simulink model "sampleModel2071"  (R2023a)
settings: Solver=VariableStepAuto  StartTime=0.0  StopTime=10.0  RelTol=1e-3
libraries: hdlsllib x7, simulink x1
settings Model: Creator=user1  LastModifiedBy=user1

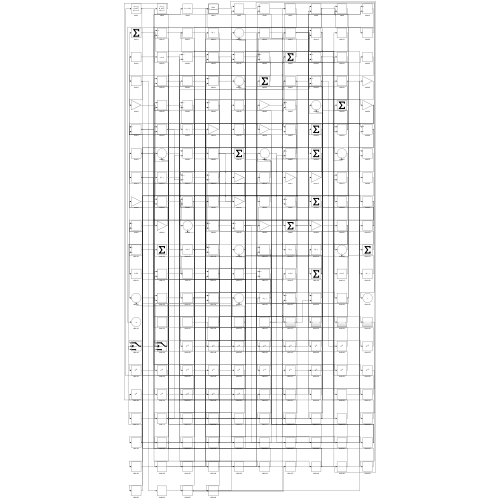
[thumbnail: Simulink's stored preview of the top-level diagram]
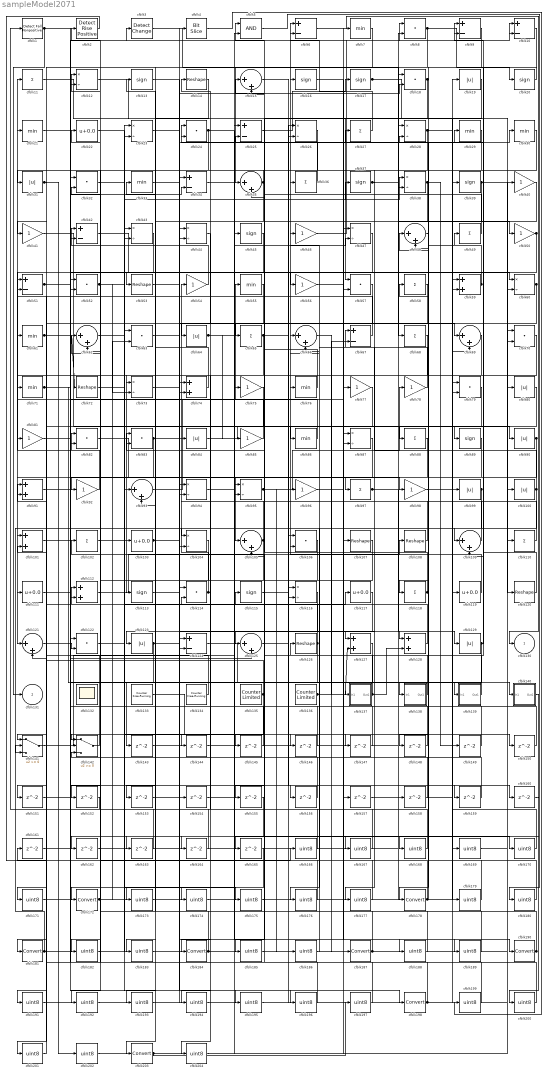
== system sampleModel2071 ==
  cfblk1 : hdlsllib/Logic and Bit Operations/Detect Fall Nonpositive  vinit=0  OutDataTypeStr=boolean
  cfblk{6,9..10,25,34,42,51,67,124} (9 alike) : Sum  Inputs=+-
  cfblk{19,31,64,80,84,90,99..100,123,129} (10 alike) : Abs  SaturateOnIntegerOverflow=off
  cfblk{59,74,91,101,112,127..128} (7 alike) : Sum
  cfblk{11,27,36,49,58,65,68,88,97,102,110,118} (12 alike) : Sum  Inputs=+
  cfblk{22,103,111,117,119} (5 alike) : Bias  Bias=0.0  SaturateOnIntegerOverflow=off
  cfblk{12,23,26,28,38,43..44,47,60,73,87,94..95,104,116} (15 alike) : Product  Inputs=*/  RndMeth=Zero  SaturateOnIntegerOverflow=on
  cfblk{15,35,48,62,66,69,93,105,109,121,125} (11 alike) : Sum  Inputs=|++
  cfblk{8,18,24,32,52,57,63,70,79,82..83,106,114,122} (14 alike) : DotProduct  OutDataTypeStr=Inherit: Inherit via internal rule
  cfblk{14,53,72,107..108,120,126} (7 alike) : Reshape
  cfblk{13,16..17,20,37,39,45,89,113,115} (10 alike) : Signum
  cfblk132 : Scope
      settings: Floating=on
  cfblk133 : hdlsllib/Sources/Counter Free-Running  NumBits=16  tsamp=-1
  cfblk134 : hdlsllib/Sources/Counter Free-Running  NumBits=16  tsamp=-1
  cfblk135 : hdlsllib/Sources/Counter Limited  uplimit=7  tsamp=-1
  cfblk136 : hdlsllib/Sources/Counter Limited  uplimit=7  tsamp=-1
  cfblk137 : Subsystem
      settings: LibrarySourceBlock=|
      | hdlsllib/Ports &
      | Subsystems/Subsystem
  cfblk138 : Subsystem
      settings: LibrarySourceBlock=|
      | hdlsllib/Ports &
      | Subsystems/Subsystem
  cfblk139 : Subsystem
      settings: LibrarySourceBlock=|
      | hdlsllib/Ports &
      | Subsystems/Subsystem
  cfblk140 : Subsystem
      settings: LibrarySourceBlock=|
      | hdlsllib/Ports &
      | Subsystems/Subsystem
  cfblk141 : Switch  SaturateOnIntegerOverflow=off  InputSameDT=off
  cfblk142 : Switch  SaturateOnIntegerOverflow=off  InputSameDT=off
  cfblk{143..165} (23 alike) : Delay  SampleTime=1
  cfblk{166..171,173..177,179..180,182..183,185..186,188..189,191..197,199..202,204} (31 alike) : DataTypeConversion  OutDataTypeStr=uint8  SaturateOnIntegerOverflow=off  RndMeth=Floor
  cfblk{172,178,181,184,187,190,198,203} (8 alike) : DataTypeConversion  SaturateOnIntegerOverflow=off  RndMeth=Floor
  cfblk2 : hdlsllib/Logic and Bit Operations/Detect Rise Positive  vinit=0  OutDataTypeStr=boolean
  cfblk{7,21,29..30,33,55,61,71,76,86} (10 alike) : MinMax
  cfblk3 : simulink/Logic and Bit Operations/Detect Change  vinit=0  OutDataTypeStr=boolean
      settings: LibrarySourceBlock=|
      | hdlsllib/Logic and Bit
      | Operations/Detect
      | Change
  cfblk4 : hdlsllib/Logic and Bit Operations/Bit Slice  lidx=7  ridx=0
  cfblk{40..41,46,50,54,56,75,77..78,81,85,92,96,98} (14 alike) : Gain
  cfblk5 : Logic  AllPortsSameDT=off  OutDataTypeStr=boolean
  cfblk130 : Outport  VectorParamsAs1DForOutWhenUnconnected=off
  cfblk131 : Outport  Port=2  VectorParamsAs1DForOutWhenUnconnected=off
  wires:
  cfblk112/1 -> cfblk108/1
  cfblk19/1 -> cfblk57/1
  cfblk129/1 -> cfblk9/2, cfblk164/1
  cfblk20/1 -> cfblk35/1
  cfblk18/1 -> cfblk118/1, cfblk65/1
  cfblk86/1 -> cfblk55/1
  cfblk90/1 -> cfblk112/1, cfblk104/2
  cfblk67/1 -> cfblk11/1
  cfblk46/1 -> cfblk8/1
  cfblk71/1 -> cfblk140/1(In1), cfblk125/2
  cfblk114/1 -> cfblk54/1, cfblk174/1
  cfblk69/1 -> cfblk113/1
  cfblk36/1 -> cfblk6/1
  cfblk95/1 -> cfblk78/1, cfblk27/1, cfblk165/1, cfblk186/1
  cfblk43/1 -> cfblk121/1
  cfblk100/1 -> cfblk38/1, cfblk109/2, cfblk67/1
  cfblk119/1 -> cfblk16/1
  cfblk45/1 -> cfblk53/1
  cfblk76/1 -> cfblk35/2
  cfblk103/1 -> cfblk34/1, cfblk18/2
  cfblk53/1 -> cfblk114/1
  cfblk123/1 -> cfblk74/1, cfblk128/1, cfblk142/2
  cfblk121/1 -> cfblk122/2
  cfblk56/1 -> cfblk30/1
  cfblk87/1 -> cfblk111/1
  cfblk28/1 -> cfblk127/1, cfblk60/1
  cfblk15/1 -> cfblk88/1
  cfblk70/1 -> cfblk181/1
  cfblk44/1 -> cfblk64/1
  cfblk66/1 -> cfblk187/1
  cfblk82/1 -> cfblk98/1
  cfblk109/1 -> cfblk58/1
  cfblk59/1 -> cfblk49/1, cfblk36/1
  cfblk8/1 -> cfblk123/1, cfblk82/2, cfblk20/1
  cfblk26/1 -> cfblk172/1
  cfblk92/1 -> cfblk21/1
  cfblk89/1 -> cfblk105/1
  cfblk27/1 -> cfblk6/2
  cfblk10/1 -> cfblk89/1
  cfblk75/1 -> cfblk203/1
  cfblk142/1 -> cfblk51/1
  cfblk42/1 -> cfblk107/1
  cfblk1/1 -> cfblk131/1, cfblk59/2
  cfblk6/1 -> cfblk130/1
  cfblk134/1 -> cfblk82/1
  cfblk35/1 -> cfblk31/1, cfblk163/1
  cfblk126/1 -> cfblk91/1, cfblk33/1, cfblk194/1
  cfblk52/1 -> cfblk93/1, cfblk73/2
  cfblk72/1 -> cfblk103/1
  cfblk64/1 -> cfblk85/1, cfblk47/2, cfblk167/1
  cfblk94/1 -> cfblk190/1
  cfblk141/1 -> cfblk45/1
  cfblk11/1 -> cfblk119/1
  cfblk47/1 -> cfblk74/2
  cfblk139/1(Out1) -> cfblk102/1
  cfblk7/1 -> cfblk41/1
  cfblk54/1 -> cfblk42/1
  cfblk41/1 -> cfblk110/1
  cfblk110/1 -> cfblk5/1
  cfblk97/1 -> cfblk10/1, cfblk129/1
  cfblk73/1 -> cfblk29/1
  cfblk60/1 -> cfblk92/1, cfblk109/1
  cfblk93/1 -> cfblk7/1
  cfblk12/1 -> cfblk80/1
  cfblk78/1 -> cfblk51/2
  cfblk39/1 -> cfblk120/1, cfblk73/1
  cfblk24/1 -> cfblk43/2, cfblk87/2
  cfblk9/1 -> cfblk138/1(In1)
  cfblk128/1 -> cfblk12/1
  cfblk83/1 -> cfblk90/1, cfblk171/1
  cfblk105/1 -> cfblk84/1, cfblk204/1
  cfblk137/1(Out1) -> cfblk96/1, cfblk128/2
  cfblk65/1 -> cfblk104/1, cfblk15/2, cfblk139/1(In1), cfblk155/1
  cfblk74/1 -> cfblk13/1
  cfblk85/1 -> cfblk61/1
  cfblk37/1 -> cfblk9/1, cfblk97/1
  cfblk106/1 -> cfblk184/1
  cfblk113/1 -> cfblk38/2
  cfblk118/1 -> cfblk15/1, cfblk83/1
  cfblk108/1 -> cfblk14/1
  cfblk17/1 -> cfblk99/1, cfblk69/2, cfblk50/1
  cfblk25/1 -> cfblk17/1
  cfblk84/1 -> cfblk86/1
  cfblk49/1 -> cfblk25/2
  cfblk136/1 -> cfblk127/2, cfblk67/2
  cfblk48/1 -> cfblk178/1
  cfblk61/1 -> cfblk72/1, cfblk95/2
  cfblk29/1 -> cfblk44/2
  cfblk32/1 -> cfblk198/1
  cfblk3/1 -> cfblk68/1
  cfblk96/1 -> cfblk47/1
  cfblk50/1 -> cfblk57/2, cfblk173/1, cfblk177/1
  cfblk124/1 -> cfblk137/1(In1)
  cfblk55/1 -> cfblk101/1
  cfblk102/1 -> cfblk37/1
  cfblk138/1(Out1) -> cfblk46/1
  cfblk104/1 -> cfblk124/2
  cfblk122/1 -> cfblk117/1
  cfblk135/1 -> cfblk142/1, cfblk91/2
  cfblk120/1 -> cfblk24/1
  cfblk21/1 -> cfblk3/1
  cfblk99/1 -> cfblk141/3, cfblk176/1
  cfblk23/1 -> cfblk4/1
  cfblk91/1 -> cfblk34/2
  cfblk51/1 -> cfblk10/2, cfblk160/1
  cfblk38/1 -> cfblk125/1, cfblk149/1
  cfblk57/1 -> cfblk141/1
  cfblk31/1 -> cfblk71/1, cfblk202/1
  cfblk13/1 -> cfblk69/1
  cfblk111/1 -> cfblk76/1
  cfblk34/1 -> cfblk56/1
  cfblk127/1 -> cfblk143/1
  cfblk143/1 -> cfblk28/1
  cfblk68/1 -> cfblk144/1
  cfblk144/1 -> cfblk5/2
  cfblk58/1 -> cfblk145/1
  cfblk145/1 -> cfblk93/2
  cfblk63/1 -> cfblk146/1
  cfblk146/1 -> cfblk25/1
  cfblk22/1 -> cfblk147/1
  cfblk147/1 -> cfblk43/1
  cfblk30/1 -> cfblk148/1
  cfblk148/1 -> cfblk44/1
  cfblk149/1 -> cfblk18/1
  cfblk125/1 -> cfblk150/1
  cfblk150/1 -> cfblk122/1
  cfblk80/1 -> cfblk151/1
  cfblk151/1 -> cfblk12/2
  cfblk107/1 -> cfblk152/1
  cfblk152/1 -> cfblk1/1
  cfblk14/1 -> cfblk153/1
  cfblk101/1 -> cfblk156/1
  cfblk156/1 -> cfblk105/2
  cfblk157/1 -> cfblk79/1
  cfblk158/1 -> cfblk142/3
  cfblk115/1 -> cfblk159/1
  cfblk159/1 -> cfblk24/2
  cfblk161/1 -> cfblk52/2
  cfblk140/1(Out1) -> cfblk162/1
  cfblk162/1 -> cfblk8/2
  cfblk163/1 -> cfblk121/2
  cfblk164/1 -> cfblk23/1
  cfblk2/1 -> cfblk166/1
  cfblk166/1 -> cfblk22/1
  cfblk167/1 -> cfblk2/1
  cfblk40/1 -> cfblk168/1
  cfblk168/1 -> cfblk114/2
  cfblk98/1 -> cfblk169/1
  cfblk169/1 -> cfblk40/1
  cfblk154/1 -> cfblk170/1
  cfblk170/1 -> cfblk59/1
  cfblk171/1 -> cfblk154/1
  cfblk172/1 -> cfblk158/1, cfblk157/1, cfblk63/2
  cfblk173/1 -> cfblk26/1
  cfblk174/1 -> cfblk26/2
  cfblk62/1 -> cfblk175/1
  cfblk175/1 -> cfblk79/2
  cfblk176/1 -> cfblk62/1
  cfblk177/1 -> cfblk62/2
  cfblk178/1 -> cfblk63/1, cfblk28/2
  cfblk133/1 -> cfblk179/1
  cfblk179/1 -> cfblk48/1
  cfblk5/1 -> cfblk180/1
  cfblk180/1 -> cfblk48/2
  cfblk181/1 -> cfblk95/1, cfblk141/2, cfblk23/2
  cfblk155/1 -> cfblk182/1
  cfblk182/1 -> cfblk70/1
  cfblk117/1 -> cfblk183/1
  cfblk183/1 -> cfblk70/2
  cfblk184/1 -> cfblk42/2, cfblk124/1
  cfblk88/1 -> cfblk185/1
  cfblk185/1 -> cfblk106/1
  cfblk186/1 -> cfblk106/2
  cfblk187/1 -> cfblk112/2, cfblk19/1
  cfblk33/1 -> cfblk188/1
  cfblk188/1 -> cfblk66/1
  cfblk16/1 -> cfblk189/1
  cfblk189/1 -> cfblk66/2
  cfblk190/1 -> cfblk83/2, cfblk87/1, cfblk126/1
  cfblk79/1 -> cfblk191/1
  cfblk191/1 -> cfblk94/1
  cfblk165/1 -> cfblk192/1
  cfblk192/1 -> cfblk94/2
  cfblk116/1 -> cfblk193/1
  cfblk193/1 -> cfblk39/1
  cfblk194/1 -> cfblk116/1
  cfblk153/1 -> cfblk195/1
  cfblk195/1 -> cfblk116/2
  cfblk81/1 -> cfblk196/1
  cfblk196/1 -> cfblk115/1
  cfblk197/1 -> cfblk81/1
  cfblk198/1 -> cfblk60/2, cfblk101/2, cfblk52/1
  cfblk4/1 -> cfblk199/1
  cfblk199/1 -> cfblk32/1
  cfblk160/1 -> cfblk200/1
  cfblk200/1 -> cfblk32/2
  cfblk77/1 -> cfblk201/1
  cfblk201/1 -> cfblk161/1
  cfblk202/1 -> cfblk77/1
  cfblk203/1 -> cfblk197/1, cfblk100/1
  cfblk204/1 -> cfblk75/1

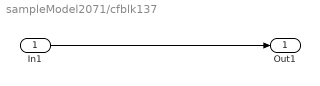
== system sampleModel2071/cfblk137 ==
  In1 : Inport
  Out1 : Outport
  wires:
  In1/1 -> Out1/1

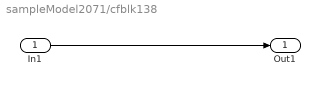
== system sampleModel2071/cfblk138 ==
  In1 : Inport
  Out1 : Outport
  wires:
  In1/1 -> Out1/1

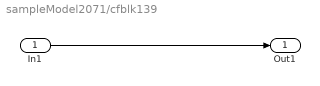
== system sampleModel2071/cfblk139 ==
  In1 : Inport
  Out1 : Outport
  wires:
  In1/1 -> Out1/1

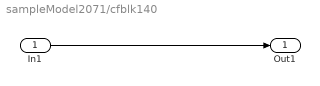
== system sampleModel2071/cfblk140 ==
  In1 : Inport
  Out1 : Outport
  wires:
  In1/1 -> Out1/1
